simulink model "full_system_parking_test"  (R2015b)
settings: Solver=ode23t  StartTime=0.0  StopTime=5  FixedStep=1  RelTol=1e-3  AbsTol=1e-6
values from neighbouring files (symbols this model uses):
  c_drag_pro = c_drag*G1.^3*r.^3/G2.^3    [Parameters.m]
  dynamic = 0.75    [Parameters.m]
  F_N = 9.8*m*weight_distribution    (= 1176)    [Parameters.m]
  G1 = 12    [Parameters.m]
  G2 = 50    [Parameters.m]
  Kt = .07329    (= 0.07329)    [Parameters.m]
  L = 4e-5    (= 4e-05)    [Parameters.m]
  N = 4    [Parameters.m]
  r = 11*.0254/2    (= 0.1397)    [Parameters.m]
  static = 1.0    (= 1)    [Parameters.m]
  T = 1/25000    (= 4e-05)    [Parameters.m]
  t1 = 1e-3    (= 0.001)    [Parameters.m]
  t2 = 1/(6*f)    (= 0.0005)    [Parameters.m]
  t3 = 3e-4    (= 0.0003)    [Parameters.m]
  viscous = 0    [Parameters.m]
undefined symbols (not defined in the file or in its folder): sigbuilder_block
libraries: fl_lib x24, nesl_utility x16, pe_lib x2, simulink x1, powerlib_meascontrol x1
settings Model: Creator=Martin Andersen  LastModifiedBy=Martin Andersen
settings SolverCC: MaxConsecutiveMinStep=10  AlgebraicLoopSolver=LineSearch

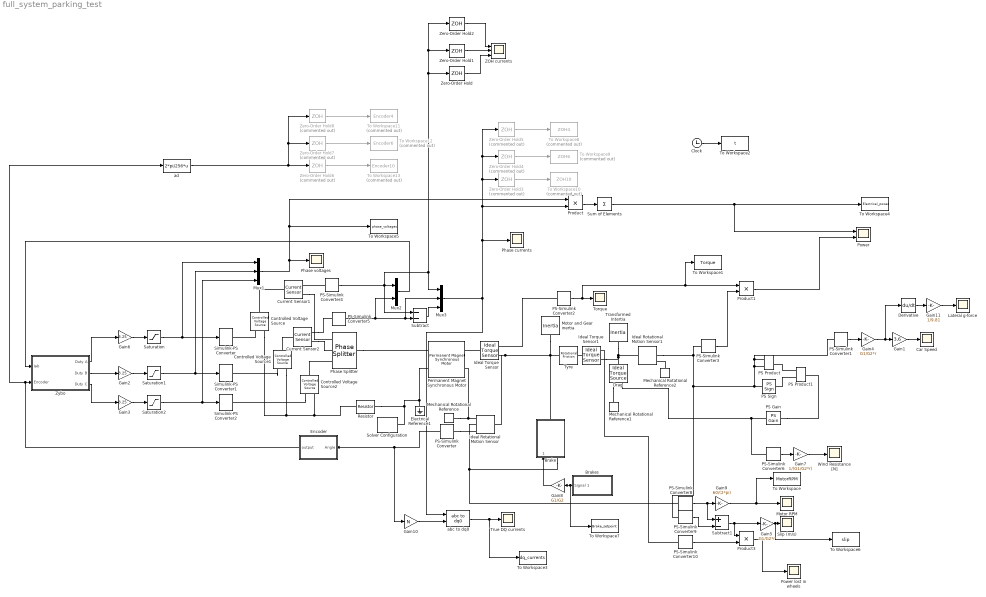
== system full_system_parking_test ==
  Brake : Subsystem
  Brakes : Subsystem  Tag=STV Subsys  LoadFcn=sigbuilder_block('load');  StartFcn=sigbuilder_block('start');  StopFcn=sigbuilder_block('stop');  ClipboardFcn=sigbuilder_block('clipboard');  mask(Sigbuilder block){}
      mask help: Simulink:masks:SigbuilderBlock_MD
      mask init:
      | if ~strcmp(get_param(bdroot(gcbh),'SimulationStatus'),'stopped') tuvar = sigbuilder_block('maskInit'); end
      settings: CopyFcn=sigbuilder_block('copy');  DeleteFcn=sigbuilder_block('delete');  ModelCloseFcn=sigbuilder_block('modelClose');  PreSaveFcn=sigbuilder_block('preSave');  PauseFcn=sigbuilder_block('pause');  ContinueFcn=sigbuilder_block('continue');  NameChangeFcn=sigbuilder_block('namechange');  OpenFcn=sigbuilder_block('open',[564 132.6 550.8 400.2 ]);  CloseFcn=sigbuilder_block('close');
      mask Display: plot(0, 0, 100, 100,[2, 2, 32, 32, 2], [68, 8, 8, 68, 68],[32, 2], [38, 38], [32, 19, 2],[53, 60, 44], [32, 17, 17, 2],[16, 16, 31, 31]);txt = getActiveGroup(gcbh);text(2, 100, txt,'verticalAlignment', 'top');
  Car Speed : Scope
  Clock : Clock
  Controlled Voltage Source : fl_lib/Electrical/Electrical Sources/Controlled Voltage Source
  Controlled Voltage Source1 : fl_lib/Electrical/Electrical Sources/Controlled Voltage Source
  Controlled Voltage Source2 : fl_lib/Electrical/Electrical Sources/Controlled Voltage Source
  Current Sensor1 : fl_lib/Electrical/Electrical Sensors/Current Sensor
  Current Sensor2 : fl_lib/Electrical/Electrical Sensors/Current Sensor
  Derivative : Derivative
  Drag : fl_lib/Mechanical/Mechanical Sources/Ideal Torque Source
  Electrical Reference1 : fl_lib/Electrical/Electrical Elements/Electrical Reference
  Encoder : Subsystem
  Gain1 : Gain  Gain=3.6
  Gain10 : Gain  Gain=N
  Gain11 : Gain  Gain=1/9.81
  Gain2 : Gain  Gain=3.25
  Gain3 : Gain  Gain=3.25
  Gain4 : Gain  Gain=G1/G2*r
  Gain5 : Gain  Gain=G1/G2*r
  Gain6 : Gain  Gain=3.25
  Gain7 : Gain  Gain=1/(G1/G2*r)
  Gain8 : Gain  Gain=G1/G2
  Gain9 : Gain  Gain=60/(2*pi)
  Ideal Rotational Motion Sensor : fl_lib/Mechanical/Mechanical Sensors/Ideal Rotational Motion Sensor  offset=0 rad
  Ideal Rotational Motion Sensor1 : fl_lib/Mechanical/Mechanical Sensors/Ideal Rotational Motion Sensor  offset=0 rad
  Ideal Torque Sensor : fl_lib/Mechanical/Mechanical Sensors/Ideal Torque Sensor
  Ideal Torque Sensor1 : fl_lib/Mechanical/Mechanical Sensors/Ideal Torque Sensor
  Lateral g-force : Scope
  Mechanical Rotational Reference : fl_lib/Mechanical/Rotational Elements/Mechanical Rotational Reference
  Mechanical Rotational Reference1 : fl_lib/Mechanical/Rotational Elements/Mechanical Rotational Reference
  Mechanical Rotational Reference2 : fl_lib/Mechanical/Rotational Elements/Mechanical Rotational Reference
  Motor RPM : Scope
  Motor and Gear inertia : fl_lib/Mechanical/Rotational Elements/Inertia  inertia=J_pro1 kg*m^2  w_specify=off  w_priority=None  w=0 rad/s  t_specify=off  t_priority=None  t=0 N*m
  Mux1 : Mux  Inputs=3
  Mux2 : Mux  Inputs=2
  Mux3 : Mux  Inputs=3
  PS Gain : fl_lib/Physical Signals/Functions/PS Gain  gain=c_drag_pro
  PS Product : fl_lib/Physical Signals/Functions/PS Product
  PS Product1 : fl_lib/Physical Signals/Functions/PS Product
  PS Sign : fl_lib/Physical Signals/Nonlinear Operators/PS Sign
  PS-Simulink Converter{,1..6,8..10} (10 alike) : nesl_utility/PS-Simulink Converter  PhysicalDomain=network_engine_domain  SubClassName=ps_output  LeftPortType=input  RightPortType=output  PseudoPeriodic=off  Frequencies=[]  Unit=1  AffineConversion=off
  Permanent Magnet Synchronous Motor : pe_lib/Machines/Permanent Magnet Rotor/Permanent Magnet Synchronous Motor  nPolePairs=N  pm_flux_linkage=Kt/N Wb  stator_param=1  Ld=L H  Lq=L H  L0=L H  Ls=L H  Lm=0 H  Ms=L/10 H  Rs=R Ohm  initial_currents=[0, 0, 0] A  axes_param=2  angular_position0=0 rad  rotor_offset=- pi / 2 rad  shift_3ph=[nan, nan, nan] rad  sqrt2OverSqrt3=nan  oneOverSqrt2=nan  twoPiOver3=nan  Lmin=1e-9 H
      settings: LogSimulationData=on
  Phase Splitter : pe_lib/Connections/Phase Splitter
  Phase currents : Scope
  Phase voltages : Scope
  Power : Scope  NumInputPorts=2
  Power lost in wheels : Scope
  Product : Product
  Product1 : Product
  Product3 : Product
  Resistor : fl_lib/Electrical/Electrical Elements/Resistor  R=1e9 Ohm  i_specify=off  i_priority=None  i=0 A  v_specify=off  v_priority=None  v=0 V
  Saturation : Saturate  UpperLimit=13.2*2*1.4  LowerLimit=-13.2*2*1.4
  Saturation1 : Saturate  UpperLimit=13.2*2*1.4  LowerLimit=-13.2*2*1.4
  Saturation2 : Saturate  UpperLimit=13.2*2*1.4  LowerLimit=-13.2*2*1.4
  Simulink-PS Converter : nesl_utility/Simulink-PS Converter  PhysicalDomain=network_engine_domain  SubClassName=ps_input  LeftPortType=input  RightPortType=output  PseudoPeriodic=off  Frequencies=[]  NoiseDistribution=none  NoiseParameters=[]  Unit=1  AffineConversion=off  InputFiltering=off  SimscapeFilterOrder=1  InputFilterTimeConstant=0.001  UdotUserProvided=1
  Simulink-PS Converter1 : nesl_utility/Simulink-PS Converter  PhysicalDomain=network_engine_domain  SubClassName=ps_input  LeftPortType=input  RightPortType=output  PseudoPeriodic=off  Frequencies=[]  NoiseDistribution=none  NoiseParameters=[]  Unit=1  AffineConversion=off  InputFiltering=off  SimscapeFilterOrder=1  InputFilterTimeConstant=0.001  UdotUserProvided=1
  Simulink-PS Converter2 : nesl_utility/Simulink-PS Converter  PhysicalDomain=network_engine_domain  SubClassName=ps_input  LeftPortType=input  RightPortType=output  PseudoPeriodic=off  Frequencies=[]  NoiseDistribution=none  NoiseParameters=[]  Unit=1  AffineConversion=off  InputFiltering=off  SimscapeFilterOrder=1  InputFilterTimeConstant=0.001  UdotUserProvided=1
  Slip (m/s) : Scope
  Solver Configuration : nesl_utility/Solver Configuration  PhysicalDomain=network_engine_domain  SubClassName=solver  LeftPortType=input  RightPortType=generic  Accelerate=off  Tones=[]  Harmonics=[]  SimulateNoise=off  Profile=off  UseLocalSampling=off  EnableSwitchedLinearOptims=on  FrequencyDomain=off  UseCCode=off  RelTol=0.001  AbsTol=1e-06  MinStep=1e-09  ToWorkspace=off  RevertToSquareIcSolve=off  NumHomotopyIterations=100  PhasorMode=off  PhasorModeNumHarmonics=1  DoDC=off  ResidualTolerance=1e-09  UseLocalSolver=off  LocalSolverChoice=NE_BACKWARD_EULER_ADVANCER  LocalSolverSampleTime=0.001  DoFixedCost=off  MaxNonlinIter=3  MaxModeIter=2  LinearAlgebra=Sparse  DelaysMemoryBudget=1024  AutomaticFiltering=on  FilteringTimeConstant=0.001
  Subtract : Sum  Inputs=--
  Subtract1 : Sum  Inputs=+-
  Sum of Elements : Sum  Inputs=+
  To Workspace : ToWorkspace  VariableName=MotorRPM  SampleTime=-1
  To Workspace1 : ToWorkspace  VariableName=Torque  SampleTime=-1
  To Workspace10 : ToWorkspace  Commented=on  VariableName=ZOH10  SampleTime=-1
  To Workspace11 : ToWorkspace  Commented=on  VariableName=Encoder4  SampleTime=-1
  To Workspace12 : ToWorkspace  Commented=on  VariableName=Encoder6  SampleTime=-1
  To Workspace13 : ToWorkspace  Commented=on  VariableName=Encoder10  SampleTime=-1
  To Workspace2 : ToWorkspace  VariableName=t  SampleTime=-1
  To Workspace3 : ToWorkspace  VariableName=dq_currents  SampleTime=-1
  To Workspace4 : ToWorkspace  VariableName=Electrical_power  SampleTime=-1
  To Workspace5 : ToWorkspace  VariableName=phase_voltages  SampleTime=-1
  To Workspace6 : ToWorkspace  VariableName=slip  SampleTime=-1
  To Workspace7 : ToWorkspace  VariableName=Brake_setpoint  SampleTime=T
      settings: Save2DSignal=2-D array (concatenate along first dimension)
  To Workspace8 : ToWorkspace  Commented=on  VariableName=ZOH4  SampleTime=-1
  To Workspace9 : ToWorkspace  Commented=on  VariableName=ZOH6  SampleTime=-1
  Torque : Scope
  Transformed Intertia : fl_lib/Mechanical/Rotational Elements/Inertia  inertia=J_pro2 kg*m^2  w_specify=off  w_priority=None  w=0 rad/s  t_specify=off  t_priority=None  t=0 N*m
  True DQ currents : Scope
  Tyre : fl_lib/Mechanical/Rotational Elements/Rotational Friction  brkwy_trq=F_N*static*r*G1/G2 N*m  Col_trq=F_N*dynamic*r*G1/G2 N*m  visc_coef=F_N*viscous*r*G1/G2 N*m/(rad/s)  trans_coef=10 s/rad  vel_thr=1e-4 rad/s  w_specify=off  w_priority=None  w=0 rad/s  t_specify=off  t_priority=None  t=0 N*m
  Wind Resistance [N] : Scope
  ZOH currents : Scope  NumInputPorts=3
  Zero-Order Hold : ZeroOrderHold  SampleTime=t3
  Zero-Order Hold1 : ZeroOrderHold  SampleTime=t2
  Zero-Order Hold2 : ZeroOrderHold  SampleTime=t1
  Zero-Order Hold3 : ZeroOrderHold  Commented=on  SampleTime=t3
  Zero-Order Hold4 : ZeroOrderHold  Commented=on  SampleTime=t2
  Zero-Order Hold5 : ZeroOrderHold  Commented=on  SampleTime=t1
  Zero-Order Hold6 : ZeroOrderHold  Commented=on  SampleTime=t3
  Zero-Order Hold7 : ZeroOrderHold  Commented=on  SampleTime=t2
  Zero-Order Hold8 : ZeroOrderHold  Commented=on  SampleTime=t1
  Zybo : Subsystem
  abc to dq0 : powerlib_meascontrol/Transformations/abc to dq0  Alignment=Aligned with phase A axis
  ad : Fcn  Expr=2*pi/256*u
  wires:
  Gain1/1 -> Car Speed/1
  PS-Simulink Converter5/1 -> Mux3/2, Subtract/2, Mux2/2
  PS-Simulink Converter6/1 -> Gain7/1
  Mux1/1 -> To Workspace5/1, Product/1, Phase voltages/1
  Mux2/1 -> Zybo/1(Iab)
  Product/1 -> Sum of Elements/1
  PS-Simulink Converter3/1 -> Product1/2
  Zybo/1(Duty A) -> Gain6/1
  PS-Simulink Converter/1 -> Gain10/1, Encoder/1(Angle)
  Encoder/1(output) -> ad/1, Zybo/2(Encoder)
  Gain6/1 -> Saturation/1
  Gain2/1 -> Saturation1/1
  Gain3/1 -> Saturation2/1
  Saturation/1 -> Mux1/1, Simulink-PS Converter/1
  Saturation1/1 -> Mux1/2, Simulink-PS Converter1/1
  Zybo/2(Duty B) -> Gain2/1
  Zybo/3(Duty C) -> Gain3/1
  Saturation2/1 -> Mux1/3, Simulink-PS Converter2/1
  Subtract/1 -> Mux3/3
  Product1/1 -> Power/2
  Brakes/1(Signal 1) -> To Workspace7/1, Gain8/1
  Gain7/1 -> Wind Resistance [N]/1
  PS-Simulink Converter9/1 -> Subtract1/2
  Subtract1/1 -> Product3/1, Gain5/1
  Gain5/1 -> To Workspace6/1, Slip (m/s)/1
  PS-Simulink Converter8/1 -> Subtract1/1, Gain9/1
  PS-Simulink Converter10/1 -> Product3/2
  Gain9/1 -> To Workspace/1, Motor RPM/1
  PS-Simulink Converter2/1 -> To Workspace1/1, Product1/1, Torque/1
  Product3/1 -> Power lost in wheels/1
  PS-Simulink Converter1/1 -> Gain4/1
  Derivative/1 -> Gain11/1
  Gain11/1 -> Lateral g-force/1
  Gain8/1 -> Brake/1(Brake torque)
  Sum of Elements/1 -> To Workspace4/1, Power/1
  Gain4/1 -> Derivative/1, Gain1/1
  Clock/1 -> To Workspace2/1
  abc to dq0/1 -> To Workspace3/1, True DQ currents/1
  Gain10/1 -> abc to dq0/2
  Zero-Order Hold2/1 -> ZOH currents/1
  Zero-Order Hold1/1 -> ZOH currents/2
  Zero-Order Hold/1 -> ZOH currents/3
  PS-Simulink Converter4/1 -> Subtract/1, Mux3/1, Zero-Order Hold2/1, Zero-Order Hold1/1, Zero-Order Hold/1, Mux2/1
  Mux3/1 -> abc to dq0/1, Phase currents/1, Zero-Order Hold5/1, Zero-Order Hold4/1, Zero-Order Hold3/1, Product/2
  ad/1 -> Zero-Order Hold7/1, Zero-Order Hold8/1, Zero-Order Hold6/1
  Zero-Order Hold5/1 -> To Workspace8/1
  Zero-Order Hold3/1 -> To Workspace10/1
  Zero-Order Hold4/1 -> To Workspace9/1
  Zero-Order Hold8/1 -> To Workspace11/1
  Zero-Order Hold7/1 -> To Workspace12/1
  Zero-Order Hold6/1 -> To Workspace13/1
  connections:
  Permanent Magnet Synchronous Motor/LConn2 -- Resistor/RConn1 -- Solver Configuration/RConn1 -- Electrical Reference1/LConn1
  Ideal Rotational Motion Sensor/RConn1 -- Mechanical Rotational Reference/LConn1 -- Permanent Magnet Synchronous Motor/RConn2
  PS-Simulink Converter3/LConn1 -- Ideal Rotational Motion Sensor1/RConn2 -- PS-Simulink Converter9/LConn1 -- PS Sign/LConn1 -- PS-Simulink Converter1/LConn1 -- PS Product/LConn1 -- PS Product/LConn2
  PS Product1/LConn2 -- PS Sign/RConn1
  PS Product1/LConn1 -- PS Product/RConn1
  PS Gain/LConn1 -- PS Product1/RConn1
  PS-Simulink Converter6/LConn1 -- Drag/RConn1 -- PS Gain/RConn1
  PS-Simulink Converter/LConn1 -- Ideal Rotational Motion Sensor/RConn3
  Controlled Voltage Source/RConn1 -- Simulink-PS Converter/RConn1
  Controlled Voltage Source1/RConn1 -- Simulink-PS Converter1/RConn1
  Controlled Voltage Source2/RConn1 -- Simulink-PS Converter2/RConn1
  Controlled Voltage Source2/LConn1 -- Phase Splitter/RConn3
  Controlled Voltage Source1/RConn2 -- Controlled Voltage Source/RConn2 -- Resistor/LConn1 -- Controlled Voltage Source2/RConn2
  Phase Splitter/LConn1 -- Permanent Magnet Synchronous Motor/LConn1
  Current Sensor1/LConn1 -- Controlled Voltage Source/LConn1
  Current Sensor1/RConn2 -- Phase Splitter/RConn1
  Current Sensor2/LConn1 -- Controlled Voltage Source1/LConn1
  Current Sensor2/RConn2 -- Phase Splitter/RConn2
  PS-Simulink Converter4/LConn1 -- Current Sensor1/RConn1
  Current Sensor2/RConn1 -- PS-Simulink Converter5/LConn1
  Drag/RConn2 -- Mechanical Rotational Reference1/LConn1
  Ideal Rotational Motion Sensor/LConn1 -- Ideal Torque Sensor/RConn1 -- Brake/RConn1 -- Motor and Gear inertia/LConn1 -- Tyre/LConn1
  PS-Simulink Converter2/LConn1 -- Ideal Torque Sensor/RConn2
  Ideal Torque Sensor/LConn1 -- Permanent Magnet Synchronous Motor/RConn1
  Drag/LConn1 -- Ideal Torque Sensor1/RConn1 -- Ideal Rotational Motion Sensor1/LConn1 -- Transformed Intertia/LConn1
  Mechanical Rotational Reference2/LConn1 -- Ideal Rotational Motion Sensor1/RConn1
  PS-Simulink Converter8/LConn1 -- Ideal Rotational Motion Sensor/RConn2 -- Brake/LConn1
  Tyre/RConn1 -- Ideal Torque Sensor1/LConn1
  PS-Simulink Converter10/LConn1 -- Ideal Torque Sensor1/RConn2

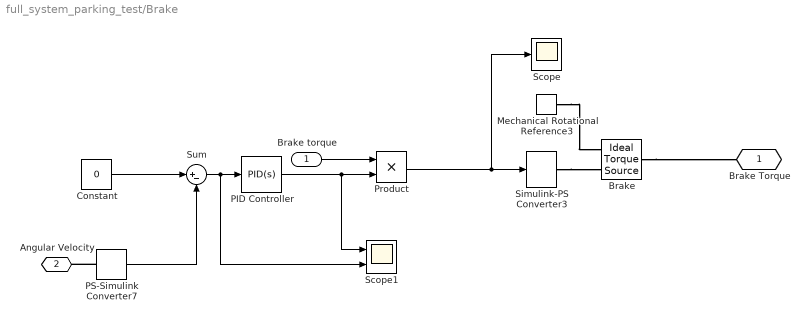
== system full_system_parking_test/Brake ==
  Brake torque : Inport
  Brake : fl_lib/Mechanical/Mechanical Sources/Ideal Torque Source
  Constant : Constant  Value=0
  Mechanical Rotational Reference3 : fl_lib/Mechanical/Rotational Elements/Mechanical Rotational Reference
  PID Controller : simulink/Continuous/PID Controller  Controller=PID  TimeDomain=Continuous-time  SampleTime=-1  IntegratorMethod=Forward Euler  FilterMethod=Forward Euler  Form=Parallel  UseFilter=on  ControllerParametersSource=internal  P=100  I=50000  D=-.1  N=100  InitialConditionSource=internal  InitialConditionForIntegrator=0  InitialConditionForFilter=0  ExternalReset=none  LimitOutput=on  UpperSaturationLimit=1  LowerSaturationLimit=-1  LinearizeAsGain=on  AntiWindupMode=back-calculation  Kb=100000  TrackingMode=off  Kt=1  PParamMin=[]  PParamMax=[]  IParamMin=[]  IParamMax=[]  DParamMin=[]  DParamMax=[]  NParamMin=[]  NParamMax=[]  KbParamMin=[]  KbParamMax=[]  KtParamMin=[]  KtParamMax=[]  POutMin=[]  POutMax=[]  IOutMin=[]  IOutMax=[]  DOutMin=[]  DOutMax=[]  NOutMin=[]  NOutMax=[]  KbOutMin=[]  KbOutMax=[]  KtOutMin=[]  KtOutMax=[]  IntegratorOutMin=[]  IntegratorOutMax=[]  FilterOutMin=[]  FilterOutMax=[]  SumOutMin=[]  SumOutMax=[]  SumI1OutMin=[]  SumI1OutMax=[]  SumI2OutMin=[]  SumI2OutMax=[]  SumI3OutMin=[]  SumI3OutMax=[]  SumDOutMin=[]  SumDOutMax=[]  SaturationOutMin=[]  SaturationOutMax=[]  IntegratorContinuousStateAttributes=''  IntegratorStateMustResolveToSignalObject=off  IntegratorRTWStateStorageClass=Auto  FilterContinuousStateAttributes=''  FilterStateMustResolveToSignalObject=off  FilterRTWStateStorageClass=Auto  DifferentiatorICPrevScaledInput=0  DifferentiatorOutMin=[]  DifferentiatorOutMax=[]
  PS-Simulink Converter7 : nesl_utility/PS-Simulink Converter  PhysicalDomain=network_engine_domain  SubClassName=ps_output  LeftPortType=input  RightPortType=output  PseudoPeriodic=off  Frequencies=[]  Unit=1  AffineConversion=off
  Product : Product
  Scope : Scope
  Scope1 : Scope  NumInputPorts=2
  Simulink-PS Converter3 : nesl_utility/Simulink-PS Converter  PhysicalDomain=network_engine_domain  SubClassName=ps_input  LeftPortType=input  RightPortType=output  PseudoPeriodic=off  Frequencies=[]  NoiseDistribution=none  NoiseParameters=[]  Unit=1  AffineConversion=off  InputFiltering=off  SimscapeFilterOrder=1  InputFilterTimeConstant=0.001  UdotUserProvided=1
  Sum : Sum  Inputs=|+-
  Brake Torque : PMIOPort  Port=1  Side=Right
  Angular Velocity : PMIOPort  Port=2  Side=Left
  wires:
  Product/1 -> Scope/1, Simulink-PS Converter3/1
  Sum/1 -> Scope1/2, PID Controller/1
  PID Controller/1 -> Scope1/1, Product/2
  Brake torque/1 -> Product/1
  Constant/1 -> Sum/1
  PS-Simulink Converter7/1 -> Sum/2
  connections:
  PS-Simulink Converter7/LConn1 -- Angular Velocity/RConn1
  Brake/LConn1 -- Brake Torque/RConn1
  Mechanical Rotational Reference3/LConn1 -- Brake/RConn2
  Simulink-PS Converter3/RConn1 -- Brake/RConn1

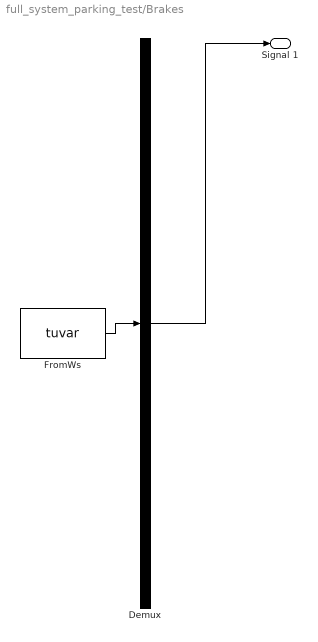
== system full_system_parking_test/Brakes ==
  Demux : Demux  Tag=STV Demux  Outputs=1
  FromWs : FromWorkspace  Tag=STV FromWs  VariableName=tuvar  SampleTime=0
      SigBuilderData=|
      | common.afterFinalStr = 'Extrapolate'
      | common.sampleTime = 0
      | dataSet.timeRange = [0 10]
      | dataSet.name = 'Group 1'
      | sbobj.Groups.Name = 'Group 1'
      | sbobj.Groups.Signals.Name = 'Signal 1'
      | sbobj.Groups.Signals.XData = [0 5.56 5.56 7.08 7.08 10]
      | sbobj.Groups.Signals.YData = [0 0 1452 1452 0 0]
  Signal 1 : Outport  Tag=STV Outport
  wires:
  Demux/1 -> Signal 1/1
  FromWs/1 -> Demux/1

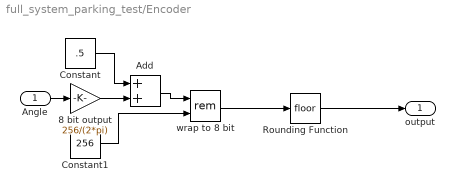
== system full_system_parking_test/Encoder ==
  Angle : Inport
  8 bit output : Gain  Gain=256/(2*pi)
  Add : Sum
  Constant : Constant  Value=.5
  Constant1 : Constant  Value=256
  Rounding Function : Rounding
  wrap to 8 bit : Math  Operator=rem  SaturateOnIntegerOverflow=on
  output : Outport
  wires:
  Constant1/1 -> wrap to 8 bit/2
  Angle/1 -> 8 bit output/1
  wrap to 8 bit/1 -> Rounding Function/1
  8 bit output/1 -> Add/2
  Add/1 -> wrap to 8 bit/1
  Constant/1 -> Add/1
  Rounding Function/1 -> output/1

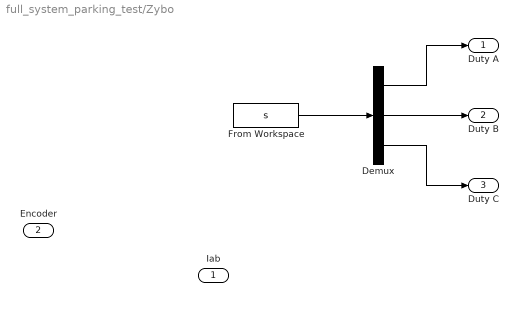
== system full_system_parking_test/Zybo ==
  Iab : Inport
  Encoder : Inport  Port=2
  Demux : Demux  Outputs=3
  From Workspace : FromWorkspace  VariableName=s  OutDataTypeStr=double  SampleTime=1
  Duty A : Outport
  Duty B : Outport  Port=2
  Duty C : Outport  Port=3
  wires:
  From Workspace/1 -> Demux/1
  Demux/1 -> Duty A/1
  Demux/2 -> Duty B/1
  Demux/3 -> Duty C/1
